simulink model "LMS02xx_realtest"  (R2018a)
settings: Solver=FixedStepDiscrete  StartTime=0.0  StopTime=inf  RelTol=1e-3
libraries: audiosources x1, dspsnks4 x1
settings Model: Creator=gianc  LastModifiedBy=gianc
settings SolverCC: AutoInsertRateTranBlk=on
settings DataIOCC: LimitDataPoints=on  SaveOutput=off  SignalLogging=off  SaveTime=off
settings OptimizationCC: LifeSpan=inf
settings DebuggingCC: AlgebraicLoopMsg=error  SingleTaskRateTransMsg=error  AllowSymbolicDim=off  SFUnexpectedBacktrackingDiag=warning  SFNoUnconditionalDefaultTransitionDiag=warning  SFExecutionAtInitializationDiag=none
settings CodeAppCC: StateflowObjectComments=on
settings GRTTargetCC: TargetLangStandard=C89/C90 (ANSI)  GeneratePreprocessorConditionals=Disable all
settings ConfigComp: CovMetricSettings=dw  CovHtmlReporting=on  CovSaveCumulativeToWorkspaceVar=on  CovSaveSingleToWorkspaceVar=on  CovExternalEMLEnable=off  CovSFcnEnable=off

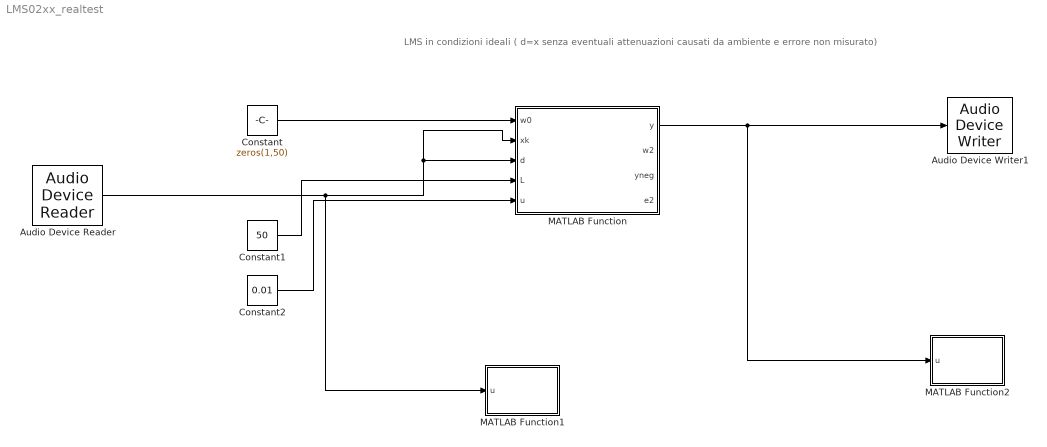
== system LMS02xx_realtest ==
  note: LMS in condizioni ideali ( d=x senza eventuali attenuazioni causati da ambiente e errore non misurato)
  Audio Device Reader : audiosources/Audio Device Reader  Driver=DirectSound  Device=Driver primario di acquisizione suoni  SampleRate=8000  NumChannels=1  SamplesPerFrame=255  BitDepth=16-bit integer  NumBuffers=10  DefaultInputChannelMapping=on  InputChannelMapping=1:2  OutputNumOverrunSamples=off  OutputDataType=double  DriverIdx=1  DeviceWarnFlag=''
      settings: SourceProductName=Audio System Toolbox  SourceProductBaseCode=AU
  Audio Device Writer1 : dspsnks4/Audio Device Writer  Driver=DirectSound  Device=Altoparlanti (Realtek High Definition Audio)  InheritSampleRate=on  SampleRate=2000  BitDepth=16-bit integer  BufferSize=4096  NumBuffers=10  DefaultOutputChannelMapping=on  OutputChannelMapping=1:2  OutputNumUnderrunSamples=off  DriverIdx=1  DeviceWarnFlag=''
  Constant : Constant  Value=zeros(1,50)  VectorParams1D=off
  Constant1 : Constant  Value=50
  Constant2 : Constant  Value=0.01
  MATLAB Function : MATLAB Function  TreatAsAtomicUnit=on
  MATLAB Function1 : MATLAB Function  TreatAsAtomicUnit=on
  MATLAB Function2 : MATLAB Function  TreatAsAtomicUnit=on
  wires:
  Constant/1 -> MATLAB Function/1(w0)
  Constant1/1 -> MATLAB Function/4(L)
  Constant2/1 -> MATLAB Function/5(u)
  Audio Device Reader/1 -> MATLAB Function1/1(u), MATLAB Function/2(xk), MATLAB Function/3(d)
  MATLAB Function/1(y) -> MATLAB Function2/1(u), Audio Device Writer1/1

== matlab function LMS02xx_realtest/MATLAB Function1 ==
  data: u input
function fcn(u)
persistent t
if isempty(t)
    t=ones(255,1);
else
    t(1)=t(255)+1;
end

for i=1:254
    t(i+1)=t(i)+1;
end

hold on
plot(t,u,'g');

end

== matlab function LMS02xx_realtest/MATLAB Function ==
  data: w0 input; y output; xk input; d input; L input; u input; w2 output; yneg output; e2 output
%y=output filter (anti noise)
%w=weights vector 1xL
%x=input vector 1xL
%xk=sampled input at time k
%d=wanted signal (ideal is x but we have d=P*x)

function [y,w2,yneg,e2] = LMS(w0,xk,d,L,u)

%global variables
[sizeD,~]=size(d);
y=zeros(sizeD,1);
yneg=zeros(sizeD,1);
alpha=0.1;
e2=zeros(sizeD,1);
persistent cnt
persistent x
persistent w

for i=1:sizeD
    
if isempty(cnt)
    cnt=1;
else
    cnt=cnt+1;
end

if isempty(x)
    x=zeros(1,L);
end

if isempty(w)
    w=w0;
end

if cnt<=L
    u=u;
else
    if cnt==L
        u = alpha/(x*(x'));
    else
        u = alpha/max(u/alpha,x*(x'));
    end
end

x=[xk(i) x(1:(L-1))]; %shift and add xk (FIFO)
y(i)= w*(x');
yneg(i)=0-y(i);
e2(i)=xk(i)-y(i);
w = w + u*x*e2(i); %refresh w for the next iteration
end
w2=w;

end

== matlab function LMS02xx_realtest/MATLAB Function2 ==
  data: u input
function fcn(u)
persistent t
if isempty(t)
    t=ones(255,1);
else
    t(1)=t(255)+1;
end

for i=1:254
    t(i+1)=t(i)+1;
end

hold on
plot(t,u,'b');

end
